simulink model "solar-panel-tracker"  (R2023a)
settings: Solver=VariableStepAuto  StartTime=0.0  StopTime=15*3600  RelTol=1e-3
undefined symbols (not defined in the file): J, Kd, Kf, Kg, Kt, L, R
libraries: slpidlib x1
settings Model: Creator=mkoda  LastModifiedBy=mkoda
settings DataIOCC: ExternalInput=[sunTime sunPosition]  LoadExternalInput=on

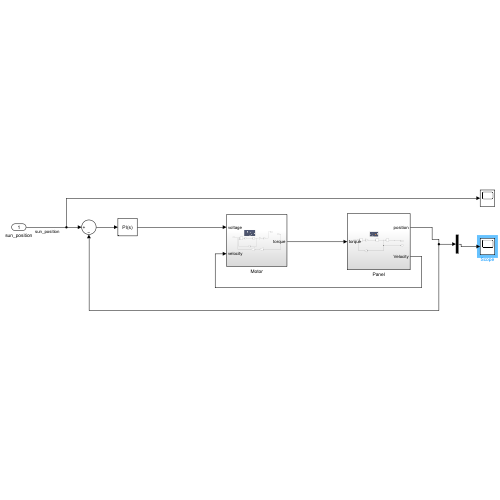
[thumbnail: Simulink's stored preview of the top-level diagram]
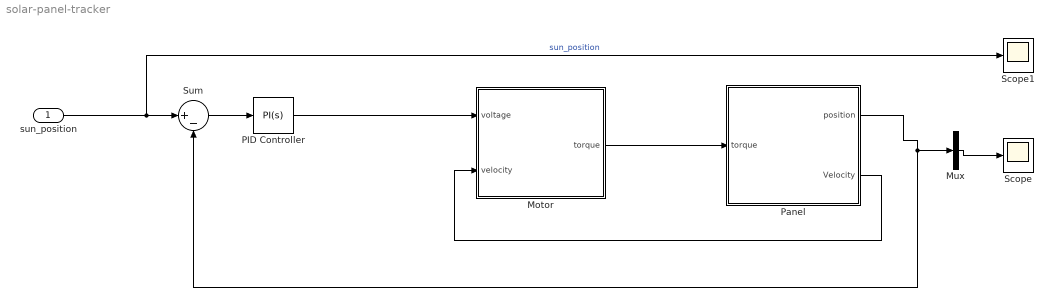
== system solar-panel-tracker ==
  sun_position : Inport
  Motor : Subsystem
  Mux : Mux  Inputs=1
  PID Controller : slpidlib/PID Controller  Controller=PI  Form=Parallel  TimeDomain=Continuous-time  UseExternalTs=off  SampleTime=-1  IntegratorMethod=Forward Euler  FilterMethod=Forward Euler  ControllerParametersSource=internal  P=240  I=180  UseKiTs=off  D=0  N=100  UseFilter=on  TunerSelectOption=Transfer Function Based (PID Tuner App)  InitialConditionSource=internal  InitialConditionForIntegrator=0  InitialConditionForFilter=0  DifferentiatorICPrevScaledInput=0  ExternalReset=none  TrackingMode=off  Kt=1  LimitOutput=off  SatLimitsSource=internal  UpperSaturationLimit=inf  LowerSaturationLimit=-inf  LinearizeAsGain=on  AntiWindupMode=none  Kb=1  LimitIntegrator=off  UpperIntegratorSaturationLimit=inf  LowerIntegratorSaturationLimit=-inf  POutMin=[]  POutMax=[]  IOutMin=[]  IOutMax=[]  DOutMin=[]  DOutMax=[]  NOutMin=[]  NOutMax=[]  SumOutMin=[]  SumOutMax=[]  SaturationOutMin=[]  SaturationOutMax=[]  PParamMin=[]  PParamMax=[]  IParamMin=[]  IParamMax=[]  DParamMin=[]  DParamMax=[]  NParamMin=[]  NParamMax=[]  KbParamMin=[]  KbParamMax=[]  KtParamMin=[]  KtParamMax=[]  KbOutMin=[]  KbOutMax=[]  KtOutMin=[]  KtOutMax=[]  IntegratorOutMin=[]  IntegratorOutMax=[]  FilterOutMin=[]  FilterOutMax=[]  SumI1OutMin=[]  SumI1OutMax=[]  SumI2OutMin=[]  SumI2OutMax=[]  SumI3OutMin=[]  SumI3OutMax=[]  SumI4OutMin=[]  SumI4OutMax=[]  SumDOutMin=[]  SumDOutMax=[]  DifferentiatorOutMin=[]  DifferentiatorOutMax=[]  FilterDiffOutCoefMin=[]  FilterDiffOutCoefMax=[]  ReciprocalOutMin=[]  ReciprocalOutMax=[]  SumDenOutMin=[]  SumDenOutMax=[]  SumNumOutMin=[]  SumNumOutMax=[]  DivideOutMin=[]  DivideOutMax=[]  UdiffTsProdOutMin=[]  UdiffTsProdOutMax=[]  NTsProdOutMin=[]  NTsProdOutMax=[]  UintegralTsProdOutMin=[]  UintegralTsProdOutMax=[]  UngainTsProdOutMin=[]  UngainTsProdOutMax=[]  ClampingZeroOutDataTypeStr=Inherit: Inherit via back propagation  ClampingZeroOutMin=[]  ClampingZeroOutMax=[]  FilterDenConstantOutDataTypeStr=Inherit: Inherit via back propagation  FilterDenConstantOutMin=[]  FilterDenConstantOutMax=[]  PCopyOutDataTypeStr=Inherit: Inherit via back propagation  PCopyOutMin=[]  PCopyOutMax=[]  NCopyOutDataTypeStr=Inherit: Inherit via back propagation  NCopyOutMin=[]  NCopyOutMax=[]  IntegratorContinuousStateAttributes=''  IntegratorStateMustResolveToSignalObject=off  IntegratorRTWStateStorageClass=Auto  FilterContinuousStateAttributes=''  FilterStateMustResolveToSignalObject=off  FilterRTWStateStorageClass=Auto  ParallelPVariant=InternalParameters  IdealPVariant=Disabled  IVariant=InternalParameters  DVariant=Disabled  IntegratorVariant=Continuous  SatVariant=Disabled  AWVariant=Passthrough  PCopyVariant=Disabled  TRVariant=Disabled  FdbkBlocksVariant=Forward  IdealPFdbkVariant=Disabled  SatFdbkVariant=Disabled  DerivativeFilterVariant=Disabled  NVariant=Disabled  NCopyVariant=Disabled_SignalSpec  FilterICVariant=Disabled  IntegratorICVariant=InternalICs  ExternalResetVariant=Disabled  TRSumVariant=Passthrough  SumFdbkVariant=Disabled  SumVariant=Sum_PI  TsampFilterVariant=InternalTs  TsampNgainVariant=Passthrough  TsampIntegralVariant=Disabled_SignalSpec  ExternalSaturationOutDataTypeStr=Inherit: Same as second input
  Panel : Subsystem
  Scope : Scope
  Scope1 : Scope
  Sum : Sum  Inputs=|+-
  wires:
  Panel/1(position) -> Sum/2, Mux/1
  Panel/2(Velocity) -> Motor/2(velocity)
  Mux/1 -> Scope/1
  PID Controller/1 -> Motor/1(voltage)
  Motor/1(torque) -> Panel/1(torque)
  sun_position/1 -> Scope1/1, Sum/1  "sun_position"
  Sum/1 -> PID Controller/1

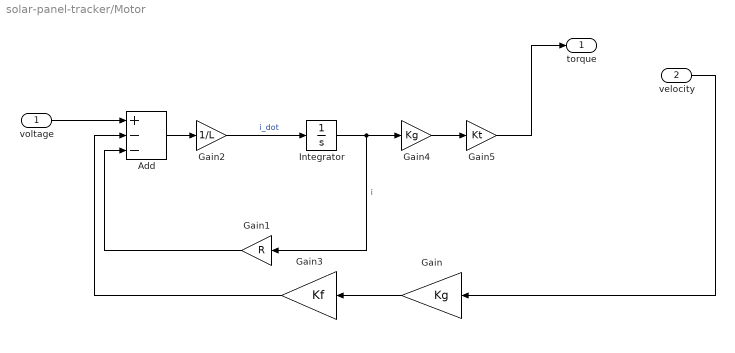
== system solar-panel-tracker/Motor ==
  voltage : Inport
  velocity : Inport  Port=2
  Add : Sum  Inputs=+--
  Gain : Gain  Gain=Kg
  Gain1 : Gain  Gain=R
  Gain2 : Gain  Gain=1/L
  Gain3 : Gain  Gain=Kf
  Gain4 : Gain  Gain=Kg
  Gain5 : Gain  Gain=Kt
  Integrator : Integrator
  torque : Outport
  wires:
  Add/1 -> Gain2/1
  Gain3/1 -> Add/2
  Integrator/1 -> Gain1/1, Gain4/1  "i"
  Gain/1 -> Gain3/1
  Gain4/1 -> Gain5/1
  Gain2/1 -> Integrator/1  "i_dot"
  Gain1/1 -> Add/3
  velocity/1 -> Gain/1
  voltage/1 -> Add/1
  Gain5/1 -> torque/1

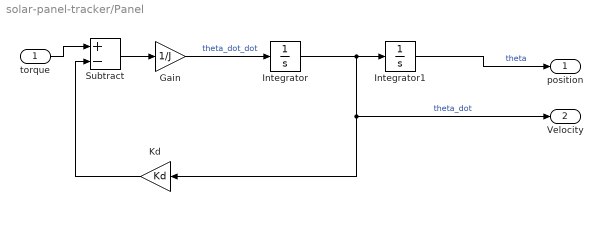
== system solar-panel-tracker/Panel ==
  torque : Inport
  Gain : Gain  Gain=1/J
  Integrator : Integrator
  Integrator1 : Integrator
  Kd : Gain  Gain=Kd
  Subtract : Sum  Inputs=+-
  position : Outport
  Velocity : Outport  Port=2
  wires:
  Integrator/1 -> Kd/1, Velocity/1, Integrator1/1  "theta_dot"
  Subtract/1 -> Gain/1
  Gain/1 -> Integrator/1  "theta_dot_dot"
  Kd/1 -> Subtract/2
  Integrator1/1 -> position/1  "theta"
  torque/1 -> Subtract/1
